simulink model "zadatak2b"  (R2023b)
settings: Solver=VariableStepAuto  StartTime=0.0  StopTime=10.0  RelTol=1e-3
settings Model: Creator=lvuke  LastModifiedBy=lvuke

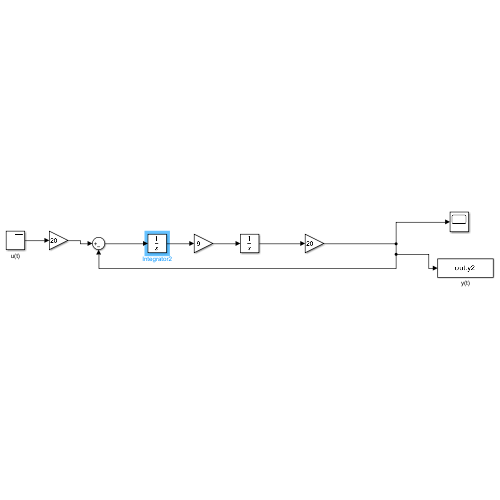
[thumbnail: Simulink's stored preview of the top-level diagram]
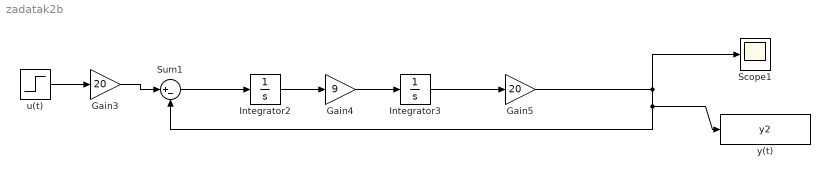
== system zadatak2b ==
  Gain3 : Gain  Gain=20
  Gain4 : Gain  Gain=9
  Gain5 : Gain  Gain=20
  Integrator2 : Integrator
  Integrator3 : Integrator
  Scope1 : Scope
  Sum1 : Sum  Inputs=|+-
  u(t) : Step  Time=5  After=3  SampleTime=0
  y(t) : ToWorkspace  VariableName=y2  SaveFormat=Timeseries  SampleTime=-1
  wires:
  u(t)/1 -> Gain3/1
  Gain3/1 -> Sum1/1
  Sum1/1 -> Integrator2/1
  Integrator2/1 -> Gain4/1
  Gain4/1 -> Integrator3/1
  Integrator3/1 -> Gain5/1
  Gain5/1 -> Sum1/2, y(t)/1, Scope1/1
